simulink library "halout"  (R2021b)
settings: Solver=VariableStepAuto  StartTime=0.0  StopTime=10.0  RelTol=1e-3
undefined symbols (not defined in the file): C_TASK_5MS_S, FALSE, KHAL_CAN1FDAPS3E2E_flg, KHAL_CAN1FDAPS3TxReq_flg, KHAL_CAN1FDVCU2E2E_flg, KHAL_CAN1FDVCU2TxReq_flg, KHAL_CAN1FDVCU3E2E_flg, KHAL_CAN1FDVCU3TxReq_flg, KHAL_CAN1TxReq_flg, KHAL_CAN2TxReq_flg, KHAL_CAN3FDVCU1TxReq_flg, KHAL_CAN3FDVCU2E2E_flg, KHAL_CAN3FDVCU2TxReq_flg, KHAL_CAN3TxReq_flg, KHAL_CAN4FDVCU1E2E_flg, KHAL_CAN4FDVCU1TxReq_flg, KHAL_CAN4TxReq_flg, KHAL_CAN5TxReq_flg, ONE_INT, TRUE, ZERO_INT
libraries: FVT_lib x383, simulink x179
(part 3 of 20)

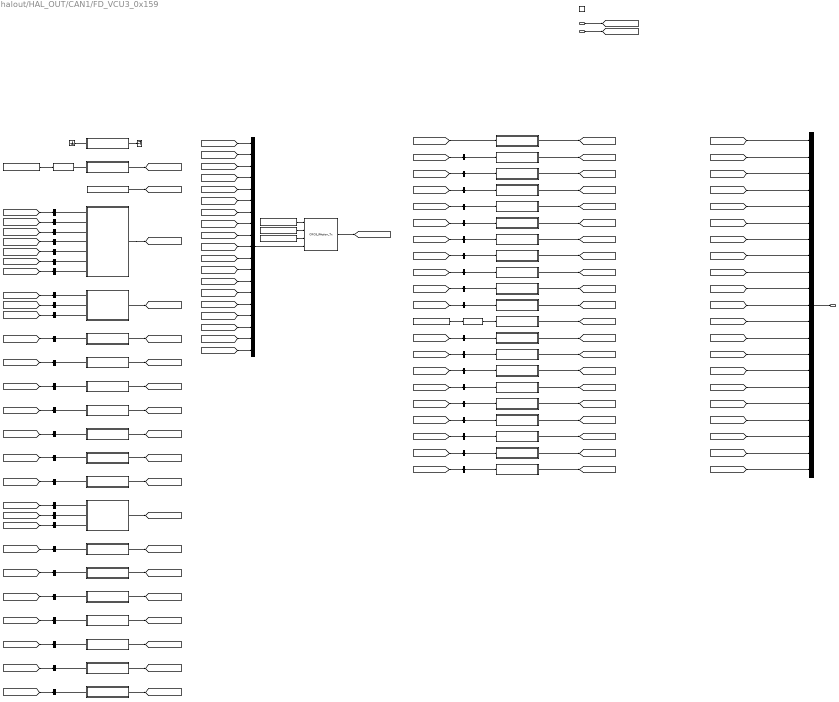
== system halout/HAL_OUT/CAN1/FD_VCU3_0x159 ==
  BSCP_outputs : Inport  OutDataTypeStr=Bus: BSCP_outputs
  BOUTP_outputs : Inport  Port=2  OutDataTypeStr=Bus: BOUTP_outputs
  Trigger : TriggerPort  TriggerType=function-call  VariantControl=(inherit)
  Byte_0 : Subsystem
  Byte_1 : Subsystem
  Byte_10 : Subsystem
  Byte_11 : Subsystem
  Byte_12 : Subsystem
  Byte_13 : Subsystem
  Byte_14 : Subsystem
  Byte_15 : Subsystem
  Byte_16 : Subsystem
  Byte_17 : Subsystem
  Byte_18 : Subsystem
  Byte_19 : Subsystem
  Byte_2 : Constant  Value=ZERO_INT
  Byte_3 : Subsystem
  Byte_4 : Subsystem
  Byte_5 : Subsystem
  Byte_6 : Subsystem
  Byte_7 : Subsystem
  Byte_8 : Subsystem
  Byte_9 : Subsystem
  CRC8_IfAction_Tx : FVT_lib/hal/CRC8_IfAction_Tx
  CSVCU3CAN1 : Subsystem
  Constant : Constant  Value=KHAL_CAN1FDVCU3E2E_flg
  Constant1 : Constant  Value=0xc8
  Constant2 : Constant  Value=0xeb
  Constant3 : Constant  Value=KHAL_CAN1FDVCU3E2E_flg
  Constant4 : Constant  Value=KHAL_CAN1FDVCU3E2E_flg
  EquivAccPedalSWSta : Subsystem
  FrEDUAvailBrkRgnTq : Subsystem
  FrEDUAvailBrkRgnTqValid : Subsystem
  FrEDURealARgnTq : Subsystem
  FrEDURealDrvOrBRgnTq : Subsystem
  FrEDUSpd : Subsystem
  FrEDUSpdValid : Subsystem
  FrRgnDecrSta : Subsystem
  FrRgnPermSta : Subsystem
  Ground : Ground
  Mux2 : Mux  Inputs=19
  PTCSPermSta : Subsystem
  RCVCU3CAN1 : Subsystem
  RgnAbnorSta : Subsystem
  RollingCounter_IfAction : FVT_lib/hal/RollingCounter_IfAction
  RollingCounter_IfAction1 : FVT_lib/hal/RollingCounter_IfAction
  RrEDUAvailBrkRgnTq : Subsystem
  RrEDUAvailBrkRgnTqValid : Subsystem
  RrEDURealARgnTq : Subsystem
  RrEDURealDrvOrBRgnTq : Subsystem
  RrEDUSpd : Subsystem
  RrEDUSpdValid : Subsystem
  RrRgnDecrSta : Subsystem
  RrRgnPermSta : Subsystem
  Terminator : Terminator
  bus_creator : BusCreator  Inputs=21  OutDataTypeStr=Bus: DT_CAN1_SG_FD_VCU3  NonVirtualBus=on
  bus_selector : BusSelector  OutputSignals=VOUTP_FrEDUSpdValid_flg
  bus_selector1 : BusSelector  OutputSignals=VOUTP_FrRgnDecrSta_flg
  bus_selector10 : BusSelector  OutputSignals=VOUTP_RrEDUSpd_rpm
  bus_selector11 : BusSelector  OutputSignals=VOUTP_RrEDURolRgnTq_Nm
  bus_selector12 : BusSelector  OutputSignals=VOUTP_RrEDURolRgnTq_Nm
  bus_selector13 : BusSelector  OutputSignals=VOUTP_RrEDUAvailBrkRgnTq_Nm
  bus_selector14 : BusSelector  OutputSignals=VOUTP_RrEDUAvailBrkRgnTq_Nm
  bus_selector15 : BusSelector  OutputSignals=VOUTP_RrEDUActTq_Nm
  bus_selector16 : BusSelector  OutputSignals=VOUTP_RrEDUActTq_Nm
  bus_selector17 : BusSelector  OutputSignals=VOUTP_FrEDUAvailBrkRgnTqV_flg
  bus_selector18 : BusSelector  OutputSignals=VOUTP_FrEDUSpd_rpm
  bus_selector19 : BusSelector  OutputSignals=VOUTP_RrEDUAvailBrkRgnTqV_flg
  bus_selector2 : BusSelector  OutputSignals=VOUTP_FrRgnPermSta_flg
  bus_selector20 : BusSelector  OutputSignals=VOUTP_FrEDUSpd_rpm
  bus_selector21 : BusSelector  OutputSignals=VOUTP_FrEDURolRgnTq_Nm
  bus_selector22 : BusSelector  OutputSignals=VOUTP_FrEDURolRgnTq_Nm
  bus_selector23 : BusSelector  OutputSignals=VOUTP_FrEDUAvailBrkRgnTq_Nm
  bus_selector24 : BusSelector  OutputSignals=VOUTP_FrEDUAvailBrkRgnTq_Nm
  bus_selector25 : BusSelector  OutputSignals=VOUTP_FrEDUActTq_Nm
  bus_selector26 : BusSelector  OutputSignals=VOUTP_FrEDUActTq_Nm
  bus_selector27 : BusSelector  OutputSignals=VOUTP_EquivAccPedalSWSta_flg
  bus_selector28 : BusSelector  OutputSignals=VOUTP_FrEDUAvailBrkRgnTq_Nm
  bus_selector29 : BusSelector  OutputSignals=VOUTP_FrEDUAvailBrkRgnTqV_flg
  bus_selector3 : BusSelector  OutputSignals=VOUTP_RgnAbnorSta_flg
  bus_selector30 : BusSelector  OutputSignals=VOUTP_FrEDURolRgnTq_Nm
  bus_selector31 : BusSelector  OutputSignals=VOUTP_FrEDUActTq_Nm
  bus_selector32 : BusSelector  OutputSignals=VOUTP_FrEDUSpd_rpm
  bus_selector33 : BusSelector  OutputSignals=VOUTP_FrEDUSpdValid_flg
  bus_selector34 : BusSelector  OutputSignals=VOUTP_FrRgnDecrSta_flg
  bus_selector35 : BusSelector  OutputSignals=VOUTP_FrRgnPermSta_flg
  bus_selector36 : BusSelector  OutputSignals=VOUTP_PTCSPermSta_flg
  bus_selector37 : BusSelector  OutputSignals=VOUTP_RgnAbnorSta_flg
  bus_selector38 : BusSelector  OutputSignals=VOUTP_RrEDUAvailBrkRgnTq_Nm
  bus_selector39 : BusSelector  OutputSignals=VOUTP_RrEDUAvailBrkRgnTqV_flg
  bus_selector4 : BusSelector  OutputSignals=VOUTP_RrEDUSpdValid_flg
  bus_selector40 : BusSelector  OutputSignals=VOUTP_RrEDURolRgnTq_Nm
  bus_selector41 : BusSelector  OutputSignals=VOUTP_RrEDUActTq_Nm
  bus_selector42 : BusSelector  OutputSignals=VOUTP_RrEDUSpd_rpm
  bus_selector43 : BusSelector  OutputSignals=VOUTP_RrEDUSpdValid_flg
  bus_selector44 : BusSelector  OutputSignals=VOUTP_RrRgnDecrSta_flg
  bus_selector45 : BusSelector  OutputSignals=VOUTP_RrRgnPermSta_flg
  bus_selector5 : BusSelector  OutputSignals=VOUTP_RrRgnDecrSta_flg
  bus_selector6 : BusSelector  OutputSignals=VOUTP_RrRgnPermSta_flg
  bus_selector7 : BusSelector  OutputSignals=VOUTP_EquivAccPedalSWSta_flg
  bus_selector8 : BusSelector  OutputSignals=VOUTP_PTCSPermSta_flg
  bus_selector9 : BusSelector  OutputSignals=VOUTP_RrEDUSpd_rpm
  FD_VCU3 : Outport
  wires:
  BSCP_outputs/1 -> [BSCP_outputs]
  BOUTP_outputs/1 -> [BOUTP_outputs]
  [CAN1_CS_VCU3_CAN1] -> bus_creator/1  "CAN1_CS_VCU3_CAN1"
  [CAN1_EquivAccPedalSWSta] -> bus_creator/2  "CAN1_EquivAccPedalSWSta"
  [CAN1_Fr_EDUAvailBrkRgnTq] -> bus_creator/3  "CAN1_Fr_EDUAvailBrkRgnTq"
  [CAN1_Fr_EDUAvailBrkRgnTqValid] -> bus_creator/4  "CAN1_Fr_EDUAvailBrkRgnTqValid"
  [CAN1_Fr_EDURealARgnTq] -> bus_creator/5  "CAN1_Fr_EDURealARgnTq"
  [CAN1_Fr_EDURealDrvOrBRgnTq] -> bus_creator/6  "CAN1_Fr_EDURealDrvOrBRgnTq"
  [CAN1_Fr_EDUSpd] -> bus_creator/7  "CAN1_Fr_EDUSpd"
  [CAN1_Fr_EDUSpdValid] -> bus_creator/8  "CAN1_Fr_EDUSpdValid"
  [CAN1_Fr_RgnDecrSta] -> bus_creator/9  "CAN1_Fr_RgnDecrSta"
  [CAN1_Fr_RgnPermSta] -> bus_creator/10  "CAN1_Fr_RgnPermSta"
  [CAN1_PTCS_PermSta] -> bus_creator/11  "CAN1_PTCS_PermSta"
  [CAN1_RC_VCU3_CAN1] -> bus_creator/12  "CAN1_RC_VCU3_CAN1"
  [CAN1_RgnAbnorSta] -> bus_creator/13  "CAN1_RgnAbnorSta"
  [CAN1_Rr_EDUAvailBrkRgnTq] -> bus_creator/14  "CAN1_Rr_EDUAvailBrkRgnTq"
  [CAN1_Rr_EDUAvailBrkRgnTqValid] -> bus_creator/15  "CAN1_Rr_EDUAvailBrkRgnTqValid"
  [CAN1_Rr_EDURealARgnTq] -> bus_creator/16  "CAN1_Rr_EDURealARgnTq"
  [CAN1_Rr_EDURealDrvOrBRgnTq] -> bus_creator/17  "CAN1_Rr_EDURealDrvOrBRgnTq"
  [CAN1_Rr_EDUSpd] -> bus_creator/18  "CAN1_Rr_EDUSpd"
  [CAN1_Rr_EDUSpdValid] -> bus_creator/19  "CAN1_Rr_EDUSpdValid"
  [CAN1_Rr_RgnDecrSta] -> bus_creator/20  "CAN1_Rr_RgnDecrSta"
  [CAN1_Rr_RgnPermSta] -> bus_creator/21  "CAN1_Rr_RgnPermSta"
  bus_creator/1 -> FD_VCU3/1
  CSVCU3CAN1/1(CAN1_CS_VCU3_CAN1) -> [CAN1_CS_VCU3_CAN1]
  EquivAccPedalSWSta/1(CAN1_EquivAccPedalSWSta) -> [CAN1_EquivAccPedalSWSta]
  FrEDUAvailBrkRgnTq/1(CAN1_Fr_EDUAvailBrkRgnTq) -> [CAN1_Fr_EDUAvailBrkRgnTq]
  FrEDUAvailBrkRgnTqValid/1(CAN1_Fr_EDUAvailBrkRgnTqValid) -> [CAN1_Fr_EDUAvailBrkRgnTqValid]
  FrEDURealARgnTq/1(CAN1_Fr_EDURealARgnTq) -> [CAN1_Fr_EDURealARgnTq]
  FrEDURealDrvOrBRgnTq/1(CAN1_Fr_EDURealDrvOrBRgnTq) -> [CAN1_Fr_EDURealDrvOrBRgnTq]
  FrEDUSpd/1(CAN1_Fr_EDUSpd) -> [CAN1_Fr_EDUSpd]
  FrEDUSpdValid/1(CAN1_Fr_EDUSpdValid) -> [CAN1_Fr_EDUSpdValid]
  FrRgnDecrSta/1(CAN1_Fr_RgnDecrSta) -> [CAN1_Fr_RgnDecrSta]
  FrRgnPermSta/1(CAN1_Fr_RgnPermSta) -> [CAN1_Fr_RgnPermSta]
  PTCSPermSta/1(CAN1_PTCS_PermSta) -> [CAN1_PTCS_PermSta]
  RCVCU3CAN1/1(CAN1_RC_VCU3_CAN1) -> [CAN1_RC_VCU3_CAN1]
  RgnAbnorSta/1(CAN1_RgnAbnorSta) -> [CAN1_RgnAbnorSta]
  RrEDUAvailBrkRgnTq/1(CAN1_Rr_EDUAvailBrkRgnTq) -> [CAN1_Rr_EDUAvailBrkRgnTq]
  RrEDUAvailBrkRgnTqValid/1(CAN1_Rr_EDUAvailBrkRgnTqValid) -> [CAN1_Rr_EDUAvailBrkRgnTqValid]
  RrEDURealARgnTq/1(CAN1_Rr_EDURealARgnTq) -> [CAN1_Rr_EDURealARgnTq]
  RrEDURealDrvOrBRgnTq/1(CAN1_Rr_EDURealDrvOrBRgnTq) -> [CAN1_Rr_EDURealDrvOrBRgnTq]
  RrEDUSpd/1(CAN1_Rr_EDUSpd) -> [CAN1_Rr_EDUSpd]
  RrEDUSpdValid/1(CAN1_Rr_EDUSpdValid) -> [CAN1_Rr_EDUSpdValid]
  RrRgnDecrSta/1(CAN1_Rr_RgnDecrSta) -> [CAN1_Rr_RgnDecrSta]
  RrRgnPermSta/1(CAN1_Rr_RgnPermSta) -> [CAN1_Rr_RgnPermSta]
  Byte_0/1(Byte_0) -> Terminator/1
  Byte_1/1(Byte_1) -> [Byte_1]
  Byte_2/1 -> [Byte_2]
  Byte_3/1(Byte_3) -> [Byte_3]
  Byte_4/1(Byte_4) -> [Byte_4]
  Byte_5/1(Byte_5) -> [Byte_5]
  Byte_6/1(Byte_6) -> [Byte_6]
  Byte_7/1(Byte_7) -> [Byte_7]
  Byte_8/1(Byte_8) -> [Byte_8]
  Byte_9/1(Byte_9) -> [Byte_9]
  Byte_10/1(Byte_10) -> [Byte_10]
  Byte_11/1(Byte_11) -> [Byte_11]
  Byte_12/1(Byte_12) -> [Byte_12]
  Byte_13/1(Byte_13) -> [Byte_13]
  Byte_14/1(Byte_14) -> [Byte_14]
  Byte_15/1(Byte_15) -> [Byte_15]
  Byte_16/1(Byte_16) -> [Byte_16]
  Byte_17/1(Byte_17) -> [Byte_17]
  Byte_18/1(Byte_18) -> [Byte_18]
  Byte_19/1(Byte_19) -> [Byte_19]
  Mux2/1 -> CRC8_IfAction_Tx/4
  Constant/1 -> CRC8_IfAction_Tx/1
  Constant1/1 -> CRC8_IfAction_Tx/2
  Constant2/1 -> CRC8_IfAction_Tx/3
  CRC8_IfAction_Tx/1 -> [CS_VCU3_CAN1]
  Ground/1 -> Byte_0/1(CS_VCU3_CAN1)
  [Byte_1] -> Mux2/1
  RollingCounter_IfAction/1 -> Byte_1/1(RC_VCU3_CAN1)
  Constant3/1 -> RollingCounter_IfAction/1
  [Byte_2] -> Mux2/2
  [Byte_3] -> Mux2/3
  bus_selector/1 -> Byte_3/1(Fr_EDUSpdValid)  "<VOUTP_FrEDUSpdValid_flg>"
  [BOUTP_outputs] -> bus_selector/1
  bus_selector1/1 -> Byte_3/2(Fr_RgnDecrSta)  "<VOUTP_FrRgnDecrSta_flg>"
  [BOUTP_outputs] -> bus_selector1/1
  bus_selector2/1 -> Byte_3/3(Fr_RgnPermSta)  "<VOUTP_FrRgnPermSta_flg>"
  [BOUTP_outputs] -> bus_selector2/1
  bus_selector3/1 -> Byte_3/4(RgnAbnorSta)  "<VOUTP_RgnAbnorSta_flg>"
  [BOUTP_outputs] -> bus_selector3/1
  bus_selector4/1 -> Byte_3/5(Rr_EDUSpdValid)  "<VOUTP_RrEDUSpdValid_flg>"
  [BOUTP_outputs] -> bus_selector4/1
  bus_selector5/1 -> Byte_3/6(Rr_RgnDecrSta)  "<VOUTP_RrRgnDecrSta_flg>"
  [BOUTP_outputs] -> bus_selector5/1
  bus_selector6/1 -> Byte_3/7(Rr_RgnPermSta)  "<VOUTP_RrRgnPermSta_flg>"
  [BOUTP_outputs] -> bus_selector6/1
  [Byte_4] -> Mux2/4
  bus_selector7/1 -> Byte_4/1(EquivAccPedalSWSta)  "<VOUTP_EquivAccPedalSWSta_flg>"
  [BOUTP_outputs] -> bus_selector7/1
  bus_selector8/1 -> Byte_4/2(PTCS_PermSta)  "<VOUTP_PTCSPermSta_flg>"
  [BOUTP_outputs] -> bus_selector8/1
  bus_selector9/1 -> Byte_4/3(Rr_EDUSpd)  "<VOUTP_RrEDUSpd_rpm>"
  [BOUTP_outputs] -> bus_selector9/1
  [Byte_5] -> Mux2/5
  bus_selector10/1 -> Byte_5/1(Rr_EDUSpd)  "<VOUTP_RrEDUSpd_rpm>"
  [BOUTP_outputs] -> bus_selector10/1
  [Byte_6] -> Mux2/6
  bus_selector11/1 -> Byte_6/1(Rr_EDURealARgnTq)  "<VOUTP_RrEDURolRgnTq_Nm>"
  [BOUTP_outputs] -> bus_selector11/1
  [Byte_7] -> Mux2/7
  bus_selector12/1 -> Byte_7/1(Rr_EDURealARgnTq)  "<VOUTP_RrEDURolRgnTq_Nm>"
  [BOUTP_outputs] -> bus_selector12/1
  [Byte_8] -> Mux2/8
  bus_selector13/1 -> Byte_8/1(Rr_EDUAvailBrkRgnTq)  "<VOUTP_RrEDUAvailBrkRgnTq_Nm>"
  [BOUTP_outputs] -> bus_selector13/1
  [Byte_9] -> Mux2/9
  bus_selector14/1 -> Byte_9/1(Rr_EDUAvailBrkRgnTq)  "<VOUTP_RrEDUAvailBrkRgnTq_Nm>"
  [BOUTP_outputs] -> bus_selector14/1
  [Byte_10] -> Mux2/10
  bus_selector15/1 -> Byte_10/1(Rr_EDURealDrvOrBRgnTq)  "<VOUTP_RrEDUActTq_Nm>"
  [BOUTP_outputs] -> bus_selector15/1
  [Byte_11] -> Mux2/11
  bus_selector16/1 -> Byte_11/1(Rr_EDURealDrvOrBRgnTq)  "<VOUTP_RrEDUActTq_Nm>"
  [BOUTP_outputs] -> bus_selector16/1
  [Byte_12] -> Mux2/12
  bus_selector17/1 -> Byte_12/1(Fr_EDUAvailBrkRgnTqValid)  "<VOUTP_FrEDUAvailBrkRgnTqV_flg>"
  [BOUTP_outputs] -> bus_selector17/1
  bus_selector18/1 -> Byte_12/2(Fr_EDUSpd)  "<VOUTP_FrEDUSpd_rpm>"
  [BOUTP_outputs] -> bus_selector18/1
  bus_selector19/1 -> Byte_12/3(Rr_EDUAvailBrkRgnTqValid)  "<VOUTP_RrEDUAvailBrkRgnTqV_flg>"
  [BOUTP_outputs] -> bus_selector19/1
  [Byte_13] -> Mux2/13
  bus_selector20/1 -> Byte_13/1(Fr_EDUSpd)  "<VOUTP_FrEDUSpd_rpm>"
  [BOUTP_outputs] -> bus_selector20/1
  [Byte_14] -> Mux2/14
  bus_selector21/1 -> Byte_14/1(Fr_EDURealARgnTq)  "<VOUTP_FrEDURolRgnTq_Nm>"
  [BOUTP_outputs] -> bus_selector21/1
  [Byte_15] -> Mux2/15
  bus_selector22/1 -> Byte_15/1(Fr_EDURealARgnTq)  "<VOUTP_FrEDURolRgnTq_Nm>"
  [BOUTP_outputs] -> bus_selector22/1
  [Byte_16] -> Mux2/16
  bus_selector23/1 -> Byte_16/1(Fr_EDUAvailBrkRgnTq)  "<VOUTP_FrEDUAvailBrkRgnTq_Nm>"
  [BOUTP_outputs] -> bus_selector23/1
  [Byte_17] -> Mux2/17
  bus_selector24/1 -> Byte_17/1(Fr_EDUAvailBrkRgnTq)  "<VOUTP_FrEDUAvailBrkRgnTq_Nm>"
  [BOUTP_outputs] -> bus_selector24/1
  [Byte_18] -> Mux2/18
  bus_selector25/1 -> Byte_18/1(Fr_EDURealDrvOrBRgnTq)  "<VOUTP_FrEDUActTq_Nm>"
  [BOUTP_outputs] -> bus_selector25/1
  [Byte_19] -> Mux2/19
  bus_selector26/1 -> Byte_19/1(Fr_EDURealDrvOrBRgnTq)  "<VOUTP_FrEDUActTq_Nm>"
  [BOUTP_outputs] -> bus_selector26/1
  [CS_VCU3_CAN1] -> CSVCU3CAN1/1(CSVCU3CAN1)
  bus_selector27/1 -> EquivAccPedalSWSta/1(EquivAccPedalSWSta)  "<VOUTP_EquivAccPedalSWSta_flg>"
  [BOUTP_outputs] -> bus_selector27/1
  bus_selector28/1 -> FrEDUAvailBrkRgnTq/1(FrEDUAvailBrkRgnTq)  "<VOUTP_FrEDUAvailBrkRgnTq_Nm>"
  [BOUTP_outputs] -> bus_selector28/1
  bus_selector29/1 -> FrEDUAvailBrkRgnTqValid/1(FrEDUAvailBrkRgnTqValid)  "<VOUTP_FrEDUAvailBrkRgnTqV_flg>"
  [BOUTP_outputs] -> bus_selector29/1
  bus_selector30/1 -> FrEDURealARgnTq/1(FrEDURealARgnTq)  "<VOUTP_FrEDURolRgnTq_Nm>"
  [BOUTP_outputs] -> bus_selector30/1
  bus_selector31/1 -> FrEDURealDrvOrBRgnTq/1(FrEDURealDrvOrBRgnTq)  "<VOUTP_FrEDUActTq_Nm>"
  [BOUTP_outputs] -> bus_selector31/1
  bus_selector32/1 -> FrEDUSpd/1(FrEDUSpd)  "<VOUTP_FrEDUSpd_rpm>"
  [BOUTP_outputs] -> bus_selector32/1
  bus_selector33/1 -> FrEDUSpdValid/1(FrEDUSpdValid)  "<VOUTP_FrEDUSpdValid_flg>"
  [BOUTP_outputs] -> bus_selector33/1
  bus_selector34/1 -> FrRgnDecrSta/1(FrRgnDecrSta)  "<VOUTP_FrRgnDecrSta_flg>"
  [BOUTP_outputs] -> bus_selector34/1
  bus_selector35/1 -> FrRgnPermSta/1(FrRgnPermSta)  "<VOUTP_FrRgnPermSta_flg>"
  [BOUTP_outputs] -> bus_selector35/1
  bus_selector36/1 -> PTCSPermSta/1(PTCSPermSta)  "<VOUTP_PTCSPermSta_flg>"
  [BOUTP_outputs] -> bus_selector36/1
  RollingCounter_IfAction1/1 -> RCVCU3CAN1/1(RCVCU3CAN1)
  Constant4/1 -> RollingCounter_IfAction1/1
  bus_selector37/1 -> RgnAbnorSta/1(RgnAbnorSta)  "<VOUTP_RgnAbnorSta_flg>"
  [BOUTP_outputs] -> bus_selector37/1
  bus_selector38/1 -> RrEDUAvailBrkRgnTq/1(RrEDUAvailBrkRgnTq)  "<VOUTP_RrEDUAvailBrkRgnTq_Nm>"
  [BOUTP_outputs] -> bus_selector38/1
  bus_selector39/1 -> RrEDUAvailBrkRgnTqValid/1(RrEDUAvailBrkRgnTqValid)  "<VOUTP_RrEDUAvailBrkRgnTqV_flg>"
  [BOUTP_outputs] -> bus_selector39/1
  bus_selector40/1 -> RrEDURealARgnTq/1(RrEDURealARgnTq)  "<VOUTP_RrEDURolRgnTq_Nm>"
  [BOUTP_outputs] -> bus_selector40/1
  bus_selector41/1 -> RrEDURealDrvOrBRgnTq/1(RrEDURealDrvOrBRgnTq)  "<VOUTP_RrEDUActTq_Nm>"
  [BOUTP_outputs] -> bus_selector41/1
  bus_selector42/1 -> RrEDUSpd/1(RrEDUSpd)  "<VOUTP_RrEDUSpd_rpm>"
  [BOUTP_outputs] -> bus_selector42/1
  bus_selector43/1 -> RrEDUSpdValid/1(RrEDUSpdValid)  "<VOUTP_RrEDUSpdValid_flg>"
  [BOUTP_outputs] -> bus_selector43/1
  bus_selector44/1 -> RrRgnDecrSta/1(RrRgnDecrSta)  "<VOUTP_RrRgnDecrSta_flg>"
  [BOUTP_outputs] -> bus_selector44/1
  bus_selector45/1 -> RrRgnPermSta/1(RrRgnPermSta)  "<VOUTP_RrRgnPermSta_flg>"
  [BOUTP_outputs] -> bus_selector45/1

== system halout/HAL_OUT/CAN1/FD_VCU3_Tx ==
  TxReq : Inport
  Chart : Stateflow chart  TreatAsAtomicUnit=on
  Constant : Constant  Value=C_TASK_5MS_S
  Constant3 : Constant  Value=CycleTime
  Data Type Conversion : DataTypeConversion  OutDataTypeStr=uint16
  Divide : Product  Inputs=*/
  Gain : Gain  Gain=0.001
  TxTrigger : Outport
  wires:
  Data Type Conversion/1 -> Chart/2(CycleCnt)
  Constant3/1 -> Gain/1
  Gain/1 -> Divide/1
  Chart/1(TxTrigger()) -> TxTrigger/1
  Divide/1 -> Data Type Conversion/1
  TxReq/1 -> Chart/1(TxReq)
  Constant/1 -> Divide/2

== system halout/HAL_OUT/CAN1/FD_VCU4_0x3C0 ==
  BSCP_outputs : Inport  OutDataTypeStr=Bus: BSCP_outputs
  BOUTP_outputs : Inport  Port=2  OutDataTypeStr=Bus: BOUTP_outputs
  EngAGSCloseSta : Subsystem
  EngActvDmpDisabSta : Subsystem
  EngCoastDwSta : Subsystem
  EngPwrLockSta : Subsystem
  Ground : Ground
  Ground1 : Ground
  Ground2 : Ground
  VehMalfunLevel : Subsystem
  bus_creator : BusCreator  Inputs=5  OutDataTypeStr=Bus: DT_CAN1_SG_FD_VCU4  NonVirtualBus=on
  bus_selector : BusSelector  OutputSignals=VOUTP_IVIPwrLockSta_enum
  bus_selector1 : BusSelector  OutputSignals=VOUTP_VehMalfunLevel_enum
  FD_VCU4 : Outport
  wires:
  BSCP_outputs/1 -> [BSCP_outputs]
  BOUTP_outputs/1 -> [BOUTP_outputs]
  [CAN1_Eng_AGSCloseSta] -> bus_creator/1  "CAN1_Eng_AGSCloseSta"
  [CAN1_Eng_ActvDmpDisabSta] -> bus_creator/2  "CAN1_Eng_ActvDmpDisabSta"
  [CAN1_Eng_CoastDwSta] -> bus_creator/3  "CAN1_Eng_CoastDwSta"
  [CAN1_Eng_PwrLockSta] -> bus_creator/4  "CAN1_Eng_PwrLockSta"
  [CAN1_VehMalfunLevel] -> bus_creator/5  "CAN1_VehMalfunLevel"
  bus_creator/1 -> FD_VCU4/1
  EngAGSCloseSta/1(CAN1_Eng_AGSCloseSta) -> [CAN1_Eng_AGSCloseSta]
  EngActvDmpDisabSta/1(CAN1_Eng_ActvDmpDisabSta) -> [CAN1_Eng_ActvDmpDisabSta]
  EngCoastDwSta/1(CAN1_Eng_CoastDwSta) -> [CAN1_Eng_CoastDwSta]
  EngPwrLockSta/1(CAN1_Eng_PwrLockSta) -> [CAN1_Eng_PwrLockSta]
  VehMalfunLevel/1(CAN1_VehMalfunLevel) -> [CAN1_VehMalfunLevel]
  Ground/1 -> EngAGSCloseSta/1(EngAGSCloseSta)
  Ground1/1 -> EngActvDmpDisabSta/1(EngActvDmpDisabSta)
  Ground2/1 -> EngCoastDwSta/1(EngCoastDwSta)
  bus_selector/1 -> EngPwrLockSta/1(EngPwrLockSta)  "<VOUTP_IVIPwrLockSta_enum>"
  [BOUTP_outputs] -> bus_selector/1
  bus_selector1/1 -> VehMalfunLevel/1(VehMalfunLevel)  "<VOUTP_VehMalfunLevel_enum>"
  [BOUTP_outputs] -> bus_selector1/1

== system halout/HAL_OUT/CAN2/FD_APS1_0x236 ==
  BSCP_outputs : Inport  OutDataTypeStr=Bus: BSCP_outputs
  BOUTP_outputs : Inport  Port=2  OutDataTypeStr=Bus: BOUTP_outputs
  APSAngleTarget : Subsystem
  APSRqEPASCtrl : Subsystem
  APSStaSystem : Subsystem
  APSVRqEPASCtrl : Subsystem
  bus_creator : BusCreator  Inputs=4  OutDataTypeStr=Bus: DT_CAN2_SG_FD_APS1  NonVirtualBus=on
  bus_selector : BusSelector  OutputSignals=VOUTP_APSAngleTarget_Deg
  bus_selector1 : BusSelector  OutputSignals=VOUTP_APSRqEPASCtrl_flg
  bus_selector2 : BusSelector  OutputSignals=VOUTP_APSStaSys_enum
  bus_selector3 : BusSelector  OutputSignals=VOUTP_APSVRqEPASCtrl_flg
  FD_APS1 : Outport
  wires:
  BSCP_outputs/1 -> [BSCP_outputs]
  BOUTP_outputs/1 -> [BOUTP_outputs]
  [CAN2_APS_Angle_Target] -> bus_creator/1  "CAN2_APS_Angle_Target"
  [CAN2_APS_Rq_EPAS_Ctrl] -> bus_creator/2  "CAN2_APS_Rq_EPAS_Ctrl"
  [CAN2_APS_Sta_System] -> bus_creator/3  "CAN2_APS_Sta_System"
  [CAN2_APS_V_Rq_EPAS_Ctrl] -> bus_creator/4  "CAN2_APS_V_Rq_EPAS_Ctrl"
  bus_creator/1 -> FD_APS1/1
  APSAngleTarget/1(CAN2_APS_Angle_Target) -> [CAN2_APS_Angle_Target]
  APSRqEPASCtrl/1(CAN2_APS_Rq_EPAS_Ctrl) -> [CAN2_APS_Rq_EPAS_Ctrl]
  APSStaSystem/1(CAN2_APS_Sta_System) -> [CAN2_APS_Sta_System]
  APSVRqEPASCtrl/1(CAN2_APS_V_Rq_EPAS_Ctrl) -> [CAN2_APS_V_Rq_EPAS_Ctrl]
  bus_selector/1 -> APSAngleTarget/1(APSAngleTarget)  "<VOUTP_APSAngleTarget_Deg>"
  [BOUTP_outputs] -> bus_selector/1
  bus_selector1/1 -> APSRqEPASCtrl/1(APSRqEPASCtrl)  "<VOUTP_APSRqEPASCtrl_flg>"
  [BOUTP_outputs] -> bus_selector1/1
  bus_selector2/1 -> APSStaSystem/1(APSStaSystem)  "<VOUTP_APSStaSys_enum>"
  [BOUTP_outputs] -> bus_selector2/1
  bus_selector3/1 -> APSVRqEPASCtrl/1(APSVRqEPASCtrl)  "<VOUTP_APSVRqEPASCtrl_flg>"
  [BOUTP_outputs] -> bus_selector3/1

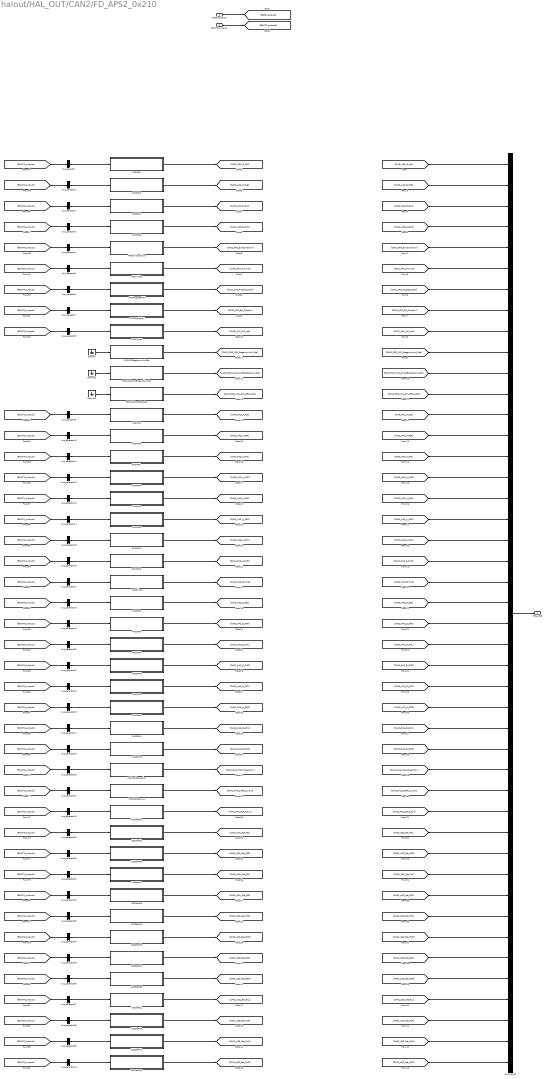
== system halout/HAL_OUT/CAN2/FD_APS2_0x210 ==
  BSCP_outputs : Inport  OutDataTypeStr=Bus: BSCP_outputs
  BOUTP_outputs : Inport  Port=2  OutDataTypeStr=Bus: BOUTP_outputs
  APSDFLL : Subsystem
  APSDFLR : Subsystem
  APSDRLL : Subsystem
  APSDRLR : Subsystem
  APSExitCondition : Subsystem
  APSHWVer : Subsystem
  APSProgressPCT : Subsystem
  APSRQDisplay : Subsystem
  APSSWVer : Subsystem
  FDCVCURegenLimIndSta : Subsystem
  FDCVCUSmartEcoSpdLimSta : Subsystem
  FDCVCUSmartEcoSta : Subsystem
  Ground : Ground
  Ground1 : Ground
  Ground2 : Ground
  PASAFCL : Subsystem
  PASAFCR : Subsystem
  PASAFML : Subsystem
  PASAFMR : Subsystem
  PASARCL : Subsystem
  PASARCR : Subsystem
  PASARML : Subsystem
  PASARMR : Subsystem
  PASChime : Subsystem
  PASDFCL : Subsystem
  PASDFCR : Subsystem
  PASDFML : Subsystem
  PASDFMR : Subsystem
  PASDRCL : Subsystem
  PASDRCR : Subsystem
  PASDRML : Subsystem
  PASDRMR : Subsystem
  PASModOperation : Subsystem
  PASSNSRLayout : Subsystem
  PASStaFSys : Subsystem
  USSStaFCL : Subsystem
  USSStaFCR : Subsystem
  USSStaFLL : Subsystem
  USSStaFLR : Subsystem
  USSStaFML : Subsystem
  USSStaFMR : Subsystem
  USSStaRCL : Subsystem
  USSStaRCR : Subsystem
  USSStaRLL : Subsystem
  USSStaRLR : Subsystem
  USSStaRML : Subsystem
  USSStaRMR : Subsystem
  bus_creator : BusCreator  Inputs=44  OutDataTypeStr=Bus: DT_CAN2_SG_FD_APS2  NonVirtualBus=on
  bus_selector : BusSelector  OutputSignals=VOUTP_APSDFLL_cm
  bus_selector1 : BusSelector  OutputSignals=VOUTP_APSDFLR_cm
  bus_selector10 : BusSelector  OutputSignals=VOUTP_PASAFCR_enum
  bus_selector11 : BusSelector  OutputSignals=VOUTP_PASAFML_enum
  bus_selector12 : BusSelector  OutputSignals=VOUTP_PASAFMR_enum
  bus_selector13 : BusSelector  OutputSignals=VOUTP_PASARCL_enum
  bus_selector14 : BusSelector  OutputSignals=VOUTP_PASARCR_enum
  bus_selector15 : BusSelector  OutputSignals=VOUTP_PASARML_enum
  bus_selector16 : BusSelector  OutputSignals=VOUTP_PASARMR_enum
  bus_selector17 : BusSelector  OutputSignals=VOUTP_Chime_enum
  bus_selector18 : BusSelector  OutputSignals=VOUTP_PASDFCL_cm
  bus_selector19 : BusSelector  OutputSignals=VOUTP_PASDFCR_cm
  bus_selector2 : BusSelector  OutputSignals=VOUTP_APSDRLL_cm
  bus_selector20 : BusSelector  OutputSignals=VOUTP_PASDFML_cm
  bus_selector21 : BusSelector  OutputSignals=VOUTP_PASDFMR_cm
  bus_selector22 : BusSelector  OutputSignals=VOUTP_PASDRCL_cm
  bus_selector23 : BusSelector  OutputSignals=VOUTP_PASDRCR_cm
  bus_selector24 : BusSelector  OutputSignals=VOUTP_PASDRML_cm
  bus_selector25 : BusSelector  OutputSignals=VOUTP_PASDRMR_cm
  bus_selector26 : BusSelector  OutputSignals=VOUTP_ModOperation_enum
  bus_selector27 : BusSelector  OutputSignals=VOUTP_SNSRLayout_enum
  bus_selector28 : BusSelector  OutputSignals=VOUTP_StaFSya_flg
  bus_selector29 : BusSelector  OutputSignals=VOUTP_USSStaFCL_flg
  bus_selector3 : BusSelector  OutputSignals=VOUTP_APSDRLR_cm
  bus_selector30 : BusSelector  OutputSignals=VOUTP_USSStaFCR_flg
  bus_selector31 : BusSelector  OutputSignals=VOUTP_USSStaFLL_flg
  bus_selector32 : BusSelector  OutputSignals=VOUTP_USSStaFLR_flg
  bus_selector33 : BusSelector  OutputSignals=VOUTP_USSStaFML_flg
  bus_selector34 : BusSelector  OutputSignals=VOUTP_USSStaFMR_flg
  bus_selector35 : BusSelector  OutputSignals=VOUTP_USSStaRCL_flg
  bus_selector36 : BusSelector  OutputSignals=VOUTP_USSStaRCR_flg
  bus_selector37 : BusSelector  OutputSignals=VOUTP_USSStaRLL_flg
  bus_selector38 : BusSelector  OutputSignals=VOUTP_USSStaRLR_flg
  bus_selector39 : BusSelector  OutputSignals=VOUTP_USSStaRML_flg
  bus_selector4 : BusSelector  OutputSignals=VOUTP_APSExitCondition_enum
  bus_selector40 : BusSelector  OutputSignals=VOUTP_USSStaRMR_flg
  bus_selector5 : BusSelector  OutputSignals=VOUTP_APSHWVer_enum
  bus_selector6 : BusSelector  OutputSignals=VOUTP_APSProgressPCT_pct
  bus_selector7 : BusSelector  OutputSignals=VOUTP_APSRQDisplay_enum
  bus_selector8 : BusSelector  OutputSignals=VOUTP_APSSWVer_enum
  bus_selector9 : BusSelector  OutputSignals=VOUTP_PASAFCL_enum
  FD_APS2 : Outport
  wires:
  BSCP_outputs/1 -> [BSCP_outputs]
  BOUTP_outputs/1 -> [BOUTP_outputs]
  [CAN2_APS_D_FLL] -> bus_creator/1  "CAN2_APS_D_FLL"
  [CAN2_APS_D_FLR] -> bus_creator/2  "CAN2_APS_D_FLR"
  [CAN2_APS_D_RLL] -> bus_creator/3  "CAN2_APS_D_RLL"
  [CAN2_APS_D_RLR] -> bus_creator/4  "CAN2_APS_D_RLR"
  [CAN2_APS_ExitCondition] -> bus_creator/5  "CAN2_APS_ExitCondition"
  [CAN2_APS_HW_Ver] -> bus_creator/6  "CAN2_APS_HW_Ver"
  [CAN2_APS_Progress_PCT] -> bus_creator/7  "CAN2_APS_Progress_PCT"
  [CAN2_APS_RQ_Display] -> bus_creator/8  "CAN2_APS_RQ_Display"
  [CAN2_APS_SW_Ver] -> bus_creator/9  "CAN2_APS_SW_Ver"
  [CAN2_FDC_VCU_RegenLimInd_Sta] -> bus_creator/10  "CAN2_FDC_VCU_RegenLimInd_Sta"
  [CAN2_FDC_VCU_SmartEcoSpdLim_Sta] -> bus_creator/11  "CAN2_FDC_VCU_SmartEcoSpdLim_Sta"
  [CAN2_FDC_VCU_SmartEco_Sta] -> bus_creator/12  "CAN2_FDC_VCU_SmartEco_Sta"
  [CAN2_PAS_A_FCL] -> bus_creator/13  "CAN2_PAS_A_FCL"
  [CAN2_PAS_A_FCR] -> bus_creator/14  "CAN2_PAS_A_FCR"
  [CAN2_PAS_A_FML] -> bus_creator/15  "CAN2_PAS_A_FML"
  [CAN2_PAS_A_FMR] -> bus_creator/16  "CAN2_PAS_A_FMR"
  [CAN2_PAS_A_RCL] -> bus_creator/17  "CAN2_PAS_A_RCL"
  [CAN2_PAS_A_RCR] -> bus_creator/18  "CAN2_PAS_A_RCR"
  [CAN2_PAS_A_RML] -> bus_creator/19  "CAN2_PAS_A_RML"
  [CAN2_PAS_A_RMR] -> bus_creator/20  "CAN2_PAS_A_RMR"
  [CAN2_PAS_Chime] -> bus_creator/21  "CAN2_PAS_Chime"
  [CAN2_PAS_D_FCL] -> bus_creator/22  "CAN2_PAS_D_FCL"
  [CAN2_PAS_D_FCR] -> bus_creator/23  "CAN2_PAS_D_FCR"
  [CAN2_PAS_D_FML] -> bus_creator/24  "CAN2_PAS_D_FML"
  [CAN2_PAS_D_FMR] -> bus_creator/25  "CAN2_PAS_D_FMR"
  [CAN2_PAS_D_RCL] -> bus_creator/26  "CAN2_PAS_D_RCL"
  [CAN2_PAS_D_RCR] -> bus_creator/27  "CAN2_PAS_D_RCR"
  [CAN2_PAS_D_RML] -> bus_creator/28  "CAN2_PAS_D_RML"
  [CAN2_PAS_D_RMR] -> bus_creator/29  "CAN2_PAS_D_RMR"
  [CAN2_PAS_Mod_Operation] -> bus_creator/30  "CAN2_PAS_Mod_Operation"
  [CAN2_PAS_SNSR_Layout] -> bus_creator/31  "CAN2_PAS_SNSR_Layout"
  [CAN2_PAS_Sta_F_Sys] -> bus_creator/32  "CAN2_PAS_Sta_F_Sys"
  [CAN2_USS_Sta_FCL] -> bus_creator/33  "CAN2_USS_Sta_FCL"
  [CAN2_USS_Sta_FCR] -> bus_creator/34  "CAN2_USS_Sta_FCR"
  [CAN2_USS_Sta_FLL] -> bus_creator/35  "CAN2_USS_Sta_FLL"
  [CAN2_USS_Sta_FLR] -> bus_creator/36  "CAN2_USS_Sta_FLR"
  [CAN2_USS_Sta_FML] -> bus_creator/37  "CAN2_USS_Sta_FML"
  [CAN2_USS_Sta_FMR] -> bus_creator/38  "CAN2_USS_Sta_FMR"
  [CAN2_USS_Sta_RCL] -> bus_creator/39  "CAN2_USS_Sta_RCL"
  [CAN2_USS_Sta_RCR] -> bus_creator/40  "CAN2_USS_Sta_RCR"
  [CAN2_USS_Sta_RLL] -> bus_creator/41  "CAN2_USS_Sta_RLL"
  [CAN2_USS_Sta_RLR] -> bus_creator/42  "CAN2_USS_Sta_RLR"
  [CAN2_USS_Sta_RML] -> bus_creator/43  "CAN2_USS_Sta_RML"
  [CAN2_USS_Sta_RMR] -> bus_creator/44  "CAN2_USS_Sta_RMR"
  bus_creator/1 -> FD_APS2/1
  APSDFLL/1(CAN2_APS_D_FLL) -> [CAN2_APS_D_FLL]
  APSDFLR/1(CAN2_APS_D_FLR) -> [CAN2_APS_D_FLR]
  APSDRLL/1(CAN2_APS_D_RLL) -> [CAN2_APS_D_RLL]
  APSDRLR/1(CAN2_APS_D_RLR) -> [CAN2_APS_D_RLR]
  APSExitCondition/1(CAN2_APS_ExitCondition) -> [CAN2_APS_ExitCondition]
  APSHWVer/1(CAN2_APS_HW_Ver) -> [CAN2_APS_HW_Ver]
  APSProgressPCT/1(CAN2_APS_Progress_PCT) -> [CAN2_APS_Progress_PCT]
  APSRQDisplay/1(CAN2_APS_RQ_Display) -> [CAN2_APS_RQ_Display]
  APSSWVer/1(CAN2_APS_SW_Ver) -> [CAN2_APS_SW_Ver]
  FDCVCURegenLimIndSta/1(CAN2_FDC_VCU_RegenLimInd_Sta) -> [CAN2_FDC_VCU_RegenLimInd_Sta]
  FDCVCUSmartEcoSpdLimSta/1(CAN2_FDC_VCU_SmartEcoSpdLim_Sta) -> [CAN2_FDC_VCU_SmartEcoSpdLim_Sta]
  FDCVCUSmartEcoSta/1(CAN2_FDC_VCU_SmartEco_Sta) -> [CAN2_FDC_VCU_SmartEco_Sta]
  PASAFCL/1(CAN2_PAS_A_FCL) -> [CAN2_PAS_A_FCL]
  PASAFCR/1(CAN2_PAS_A_FCR) -> [CAN2_PAS_A_FCR]
  PASAFML/1(CAN2_PAS_A_FML) -> [CAN2_PAS_A_FML]
  PASAFMR/1(CAN2_PAS_A_FMR) -> [CAN2_PAS_A_FMR]
  PASARCL/1(CAN2_PAS_A_RCL) -> [CAN2_PAS_A_RCL]
  PASARCR/1(CAN2_PAS_A_RCR) -> [CAN2_PAS_A_RCR]
  PASARML/1(CAN2_PAS_A_RML) -> [CAN2_PAS_A_RML]
  PASARMR/1(CAN2_PAS_A_RMR) -> [CAN2_PAS_A_RMR]
  PASChime/1(CAN2_PAS_Chime) -> [CAN2_PAS_Chime]
  PASDFCL/1(CAN2_PAS_D_FCL) -> [CAN2_PAS_D_FCL]
  PASDFCR/1(CAN2_PAS_D_FCR) -> [CAN2_PAS_D_FCR]
  PASDFML/1(CAN2_PAS_D_FML) -> [CAN2_PAS_D_FML]
  PASDFMR/1(CAN2_PAS_D_FMR) -> [CAN2_PAS_D_FMR]
  PASDRCL/1(CAN2_PAS_D_RCL) -> [CAN2_PAS_D_RCL]
  PASDRCR/1(CAN2_PAS_D_RCR) -> [CAN2_PAS_D_RCR]
  PASDRML/1(CAN2_PAS_D_RML) -> [CAN2_PAS_D_RML]
  PASDRMR/1(CAN2_PAS_D_RMR) -> [CAN2_PAS_D_RMR]
  PASModOperation/1(CAN2_PAS_Mod_Operation) -> [CAN2_PAS_Mod_Operation]
  PASSNSRLayout/1(CAN2_PAS_SNSR_Layout) -> [CAN2_PAS_SNSR_Layout]
  PASStaFSys/1(CAN2_PAS_Sta_F_Sys) -> [CAN2_PAS_Sta_F_Sys]
  USSStaFCL/1(CAN2_USS_Sta_FCL) -> [CAN2_USS_Sta_FCL]
  USSStaFCR/1(CAN2_USS_Sta_FCR) -> [CAN2_USS_Sta_FCR]
  USSStaFLL/1(CAN2_USS_Sta_FLL) -> [CAN2_USS_Sta_FLL]
  USSStaFLR/1(CAN2_USS_Sta_FLR) -> [CAN2_USS_Sta_FLR]
  USSStaFML/1(CAN2_USS_Sta_FML) -> [CAN2_USS_Sta_FML]
  USSStaFMR/1(CAN2_USS_Sta_FMR) -> [CAN2_USS_Sta_FMR]
  USSStaRCL/1(CAN2_USS_Sta_RCL) -> [CAN2_USS_Sta_RCL]
  USSStaRCR/1(CAN2_USS_Sta_RCR) -> [CAN2_USS_Sta_RCR]
  USSStaRLL/1(CAN2_USS_Sta_RLL) -> [CAN2_USS_Sta_RLL]
  USSStaRLR/1(CAN2_USS_Sta_RLR) -> [CAN2_USS_Sta_RLR]
  USSStaRML/1(CAN2_USS_Sta_RML) -> [CAN2_USS_Sta_RML]
  USSStaRMR/1(CAN2_USS_Sta_RMR) -> [CAN2_USS_Sta_RMR]
  bus_selector/1 -> APSDFLL/1(APSDFLL)  "<VOUTP_APSDFLL_cm>"
  [BOUTP_outputs] -> bus_selector/1
  bus_selector1/1 -> APSDFLR/1(APSDFLR)  "<VOUTP_APSDFLR_cm>"
  [BOUTP_outputs] -> bus_selector1/1
  bus_selector2/1 -> APSDRLL/1(APSDRLL)  "<VOUTP_APSDRLL_cm>"
  [BOUTP_outputs] -> bus_selector2/1
  bus_selector3/1 -> APSDRLR/1(APSDRLR)  "<VOUTP_APSDRLR_cm>"
  [BOUTP_outputs] -> bus_selector3/1
  bus_selector4/1 -> APSExitCondition/1(APSExitCondition)  "<VOUTP_APSExitCondition_enum>"
  [BOUTP_outputs] -> bus_selector4/1
  bus_selector5/1 -> APSHWVer/1(APSHWVer)  "<VOUTP_APSHWVer_enum>"
  [BOUTP_outputs] -> bus_selector5/1
  bus_selector6/1 -> APSProgressPCT/1(APSProgressPCT)  "<VOUTP_APSProgressPCT_pct>"
  [BOUTP_outputs] -> bus_selector6/1
  bus_selector7/1 -> APSRQDisplay/1(APSRQDisplay)  "<VOUTP_APSRQDisplay_enum>"
  [BOUTP_outputs] -> bus_selector7/1
  bus_selector8/1 -> APSSWVer/1(APSSWVer)  "<VOUTP_APSSWVer_enum>"
  [BOUTP_outputs] -> bus_selector8/1
  Ground/1 -> FDCVCURegenLimIndSta/1(FDCVCURegenLimIndSta)
  Ground1/1 -> FDCVCUSmartEcoSpdLimSta/1(FDCVCUSmartEcoSpdLimSta)
  Ground2/1 -> FDCVCUSmartEcoSta/1(FDCVCUSmartEcoSta)
  bus_selector9/1 -> PASAFCL/1(PASAFCL)  "<VOUTP_PASAFCL_enum>"
  [BOUTP_outputs] -> bus_selector9/1
  bus_selector10/1 -> PASAFCR/1(PASAFCR)  "<VOUTP_PASAFCR_enum>"
  [BOUTP_outputs] -> bus_selector10/1
  bus_selector11/1 -> PASAFML/1(PASAFML)  "<VOUTP_PASAFML_enum>"
  [BOUTP_outputs] -> bus_selector11/1
  bus_selector12/1 -> PASAFMR/1(PASAFMR)  "<VOUTP_PASAFMR_enum>"
  [BOUTP_outputs] -> bus_selector12/1
  bus_selector13/1 -> PASARCL/1(PASARCL)  "<VOUTP_PASARCL_enum>"
  [BOUTP_outputs] -> bus_selector13/1
  bus_selector14/1 -> PASARCR/1(PASARCR)  "<VOUTP_PASARCR_enum>"
  [BOUTP_outputs] -> bus_selector14/1
  bus_selector15/1 -> PASARML/1(PASARML)  "<VOUTP_PASARML_enum>"
  [BOUTP_outputs] -> bus_selector15/1
  bus_selector16/1 -> PASARMR/1(PASARMR)  "<VOUTP_PASARMR_enum>"
  [BOUTP_outputs] -> bus_selector16/1
  bus_selector17/1 -> PASChime/1(PASChime)  "<VOUTP_Chime_enum>"
  [BOUTP_outputs] -> bus_selector17/1
  bus_selector18/1 -> PASDFCL/1(PASDFCL)  "<VOUTP_PASDFCL_cm>"
  [BOUTP_outputs] -> bus_selector18/1
  bus_selector19/1 -> PASDFCR/1(PASDFCR)  "<VOUTP_PASDFCR_cm>"
  [BOUTP_outputs] -> bus_selector19/1
  bus_selector20/1 -> PASDFML/1(PASDFML)  "<VOUTP_PASDFML_cm>"
  [BOUTP_outputs] -> bus_selector20/1
  bus_selector21/1 -> PASDFMR/1(PASDFMR)  "<VOUTP_PASDFMR_cm>"
  [BOUTP_outputs] -> bus_selector21/1
  bus_selector22/1 -> PASDRCL/1(PASDRCL)  "<VOUTP_PASDRCL_cm>"
  [BOUTP_outputs] -> bus_selector22/1
  bus_selector23/1 -> PASDRCR/1(PASDRCR)  "<VOUTP_PASDRCR_cm>"
  [BOUTP_outputs] -> bus_selector23/1
  bus_selector24/1 -> PASDRML/1(PASDRML)  "<VOUTP_PASDRML_cm>"
  [BOUTP_outputs] -> bus_selector24/1
  bus_selector25/1 -> PASDRMR/1(PASDRMR)  "<VOUTP_PASDRMR_cm>"
  [BOUTP_outputs] -> bus_selector25/1
  bus_selector26/1 -> PASModOperation/1(PASModOperation)  "<VOUTP_ModOperation_enum>"
  [BOUTP_outputs] -> bus_selector26/1
  bus_selector27/1 -> PASSNSRLayout/1(PASSNSRLayout)  "<VOUTP_SNSRLayout_enum>"
  [BOUTP_outputs] -> bus_selector27/1
  bus_selector28/1 -> PASStaFSys/1(PASStaFSys)  "<VOUTP_StaFSya_flg>"
  [BOUTP_outputs] -> bus_selector28/1
  bus_selector29/1 -> USSStaFCL/1(USSStaFCL)  "<VOUTP_USSStaFCL_flg>"
  [BOUTP_outputs] -> bus_selector29/1
  bus_selector30/1 -> USSStaFCR/1(USSStaFCR)  "<VOUTP_USSStaFCR_flg>"
  [BOUTP_outputs] -> bus_selector30/1
  bus_selector31/1 -> USSStaFLL/1(USSStaFLL)  "<VOUTP_USSStaFLL_flg>"
  [BOUTP_outputs] -> bus_selector31/1
  bus_selector32/1 -> USSStaFLR/1(USSStaFLR)  "<VOUTP_USSStaFLR_flg>"
  [BOUTP_outputs] -> bus_selector32/1
  bus_selector33/1 -> USSStaFML/1(USSStaFML)  "<VOUTP_USSStaFML_flg>"
  [BOUTP_outputs] -> bus_selector33/1
  bus_selector34/1 -> USSStaFMR/1(USSStaFMR)  "<VOUTP_USSStaFMR_flg>"
  [BOUTP_outputs] -> bus_selector34/1
  bus_selector35/1 -> USSStaRCL/1(USSStaRCL)  "<VOUTP_USSStaRCL_flg>"
  [BOUTP_outputs] -> bus_selector35/1
  bus_selector36/1 -> USSStaRCR/1(USSStaRCR)  "<VOUTP_USSStaRCR_flg>"
  [BOUTP_outputs] -> bus_selector36/1
  bus_selector37/1 -> USSStaRLL/1(USSStaRLL)  "<VOUTP_USSStaRLL_flg>"
  [BOUTP_outputs] -> bus_selector37/1
  bus_selector38/1 -> USSStaRLR/1(USSStaRLR)  "<VOUTP_USSStaRLR_flg>"
  [BOUTP_outputs] -> bus_selector38/1
  bus_selector39/1 -> USSStaRML/1(USSStaRML)  "<VOUTP_USSStaRML_flg>"
  [BOUTP_outputs] -> bus_selector39/1
  bus_selector40/1 -> USSStaRMR/1(USSStaRMR)  "<VOUTP_USSStaRMR_flg>"
  [BOUTP_outputs] -> bus_selector40/1

== system halout/HAL_OUT/CAN2/FD_APS3_0x238 ==
  BSCP_outputs : Inport  OutDataTypeStr=Bus: BSCP_outputs
  BOUTP_outputs : Inport  Port=2  OutDataTypeStr=Bus: BOUTP_outputs
  APS3LifeCount : Subsystem
  APS3checksum : Subsystem
  APSDecReq : Subsystem
  APSDecReqA : Subsystem
  APSOpenPTG : Subsystem
  APSReq : Subsystem
  CAASSta : Subsystem
  Ground : Ground
  Ground1 : Ground
  Ground2 : Ground
  SPTGDet : Subsystem
  SPTGSta : Subsystem
  bus_creator : BusCreator  Inputs=9  OutDataTypeStr=Bus: DT_CAN2_SG_FD_APS3  NonVirtualBus=on
  bus_selector : BusSelector  OutputSignals=VOUTP_APSOpenPTG_flg
  bus_selector1 : BusSelector  OutputSignals=VOUTP_APSDecReq_mps2
  bus_selector2 : BusSelector  OutputSignals=VOUTP_APSDecReqA_flg
  bus_selector3 : BusSelector  OutputSignals=VOUTP_APSReq_enum
  bus_selector4 : BusSelector  OutputSignals=VOUTP_CAASSta_enum
  bus_selector5 : BusSelector  OutputSignals=VOUTP_SPTGDet_flg
  FD_APS3 : Outport
  wires:
  BSCP_outputs/1 -> [BSCP_outputs]
  BOUTP_outputs/1 -> [BOUTP_outputs]
  [CAN2_APS3_LifeCount] -> bus_creator/1  "CAN2_APS3_LifeCount"
  [CAN2_APS3_checksum] -> bus_creator/2  "CAN2_APS3_checksum"
  [CAN2_APSOpenPTG] -> bus_creator/3  "CAN2_APSOpenPTG"
  [CAN2_APS_DecReq] -> bus_creator/4  "CAN2_APS_DecReq"
  [CAN2_APS_DecReq_A] -> bus_creator/5  "CAN2_APS_DecReq_A"
  [CAN2_APS_Req] -> bus_creator/6  "CAN2_APS_Req"
  [CAN2_CAAS_Sta] -> bus_creator/7  "CAN2_CAAS_Sta"
  [CAN2_SPTGDet] -> bus_creator/8  "CAN2_SPTGDet"
  [CAN2_SPTG_Sta] -> bus_creator/9  "CAN2_SPTG_Sta"
  bus_creator/1 -> FD_APS3/1
  APS3LifeCount/1(CAN2_APS3_LifeCount) -> [CAN2_APS3_LifeCount]
  APS3checksum/1(CAN2_APS3_checksum) -> [CAN2_APS3_checksum]
  APSOpenPTG/1(CAN2_APSOpenPTG) -> [CAN2_APSOpenPTG]
  APSDecReq/1(CAN2_APS_DecReq) -> [CAN2_APS_DecReq]
  APSDecReqA/1(CAN2_APS_DecReq_A) -> [CAN2_APS_DecReq_A]
  APSReq/1(CAN2_APS_Req) -> [CAN2_APS_Req]
  CAASSta/1(CAN2_CAAS_Sta) -> [CAN2_CAAS_Sta]
  SPTGDet/1(CAN2_SPTGDet) -> [CAN2_SPTGDet]
  SPTGSta/1(CAN2_SPTG_Sta) -> [CAN2_SPTG_Sta]
  Ground/1 -> APS3LifeCount/1(APS3LifeCount)
  Ground1/1 -> APS3checksum/1(APS3checksum)
  bus_selector/1 -> APSOpenPTG/1(APSOpenPTG)  "<VOUTP_APSOpenPTG_flg>"
  [BOUTP_outputs] -> bus_selector/1
  bus_selector1/1 -> APSDecReq/1(APSDecReq)  "<VOUTP_APSDecReq_mps2>"
  [BOUTP_outputs] -> bus_selector1/1
  bus_selector2/1 -> APSDecReqA/1(APSDecReqA)  "<VOUTP_APSDecReqA_flg>"
  [BOUTP_outputs] -> bus_selector2/1
  bus_selector3/1 -> APSReq/1(APSReq)  "<VOUTP_APSReq_enum>"
  [BOUTP_outputs] -> bus_selector3/1
  bus_selector4/1 -> CAASSta/1(CAASSta)  "<VOUTP_CAASSta_enum>"
  [BOUTP_outputs] -> bus_selector4/1
  bus_selector5/1 -> SPTGDet/1(SPTGDet)  "<VOUTP_SPTGDet_flg>"
  [BOUTP_outputs] -> bus_selector5/1
  Ground2/1 -> SPTGSta/1(SPTGSta)
